simulink model "engineMassModel2"  (R2020a)
settings: Solver=VariableStepAuto  StartTime=0.0  StopTime=30  RelTol=1e-3
values from neighbouring files (symbols this model uses):
  average_rho = (LOX_rho*LOX_l + fuel_rho*fuel_l)/(LOX_l+fuel_l)    (= 1.00923076923)    [engineMassModelM.m]
  CdA = mdot_i/(sqrt(2*(p_i-14.7)))    [engineMassModelM.m]
  m_i = 1.09769264    [engineMassModelM.m]
  mil_to_cu_in = 0.0610237    [engineMassModelM.m]
  p_i = 1000    [engineMassModelM.m]
  press_vol = press_l * pi() * (tube_id/2)^2    [engineMassModelM.m]
settings Model: Creator=Makar  LastModifiedBy=Makar

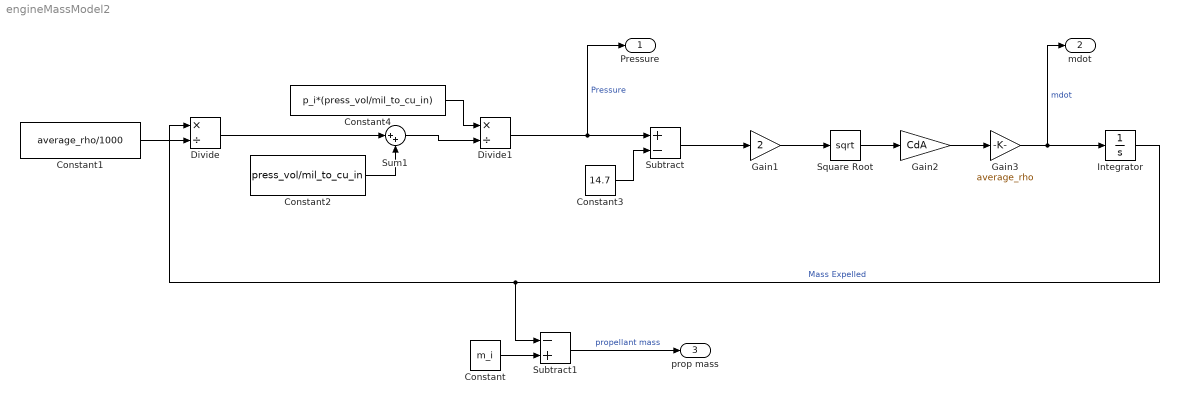
== system engineMassModel2 ==
  Constant : Constant  Value=m_i
  Constant1 : Constant  Value=average_rho/1000
  Constant2 : Constant  Value=press_vol/mil_to_cu_in
  Constant3 : Constant  Value=14.7
  Constant4 : Constant  Value=p_i*(press_vol/mil_to_cu_in)
  Divide : Product  Inputs=*/
  Divide1 : Product  Inputs=*/
  Gain1 : Gain  Gain=2
  Gain2 : Gain  Gain=CdA
  Gain3 : Gain  Gain=average_rho
  Integrator : Integrator
  Square Root : Sqrt  SaturateOnIntegerOverflow=on
  Subtract : Sum  Inputs=+-
  Subtract1 : Sum  Inputs=-+
  Sum1 : Sum  Inputs=|++
  Pressure : Outport  SignalName=Pressure
  mdot : Outport  Port=2  SignalName=mdot
  prop mass : Outport  Port=3  SignalName=prop mass
  wires:
  Constant1/1 -> Divide/2
  Divide/1 -> Sum1/1
  Constant2/1 -> Sum1/2
  Divide1/1 -> Pressure/1, Subtract/1  "Pressure"
  Constant3/1 -> Subtract/2
  Subtract/1 -> Gain1/1
  Gain1/1 -> Square Root/1
  Square Root/1 -> Gain2/1
  Gain2/1 -> Gain3/1
  Gain3/1 -> mdot/1, Integrator/1  "mdot"
  Integrator/1 -> Subtract1/1, Divide/1  "Mass Expelled"
  Sum1/1 -> Divide1/2
  Constant4/1 -> Divide1/1
  Constant/1 -> Subtract1/2
  Subtract1/1 -> prop mass/1  "propellant mass"
